simulink model "TP4_control_linealizante_Haldane_params_desconocidos_int"  (R2024b)
settings: Solver=VariableStepAuto  StartTime=0.0  StopTime=10.0  FixedStep=0.  RelTol=1e-3
values from neighbouring files (symbols this model uses):
  e0 = mu_r*1.5    (= 0.12675)    [Main_entregable.m]
  states0 = [x0;s0]*1.5    [DatosModeloTP4.m]    (also in Main_entregable.m = [x0;s0;0;0]*1.5)
  v0 = 1    [DatosModeloTP4.m]
settings Model: Creator=tomii  LastModifiedBy=tomii

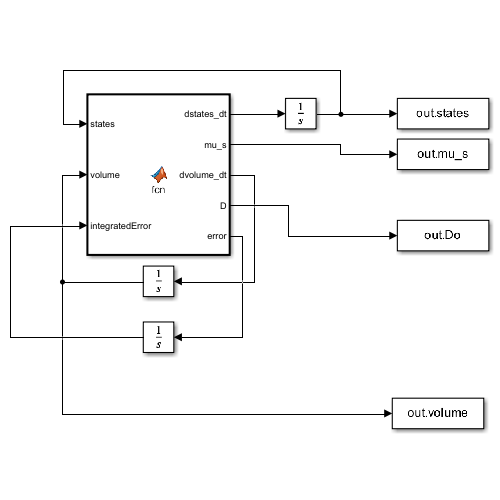
[thumbnail: Simulink's stored preview of the top-level diagram]
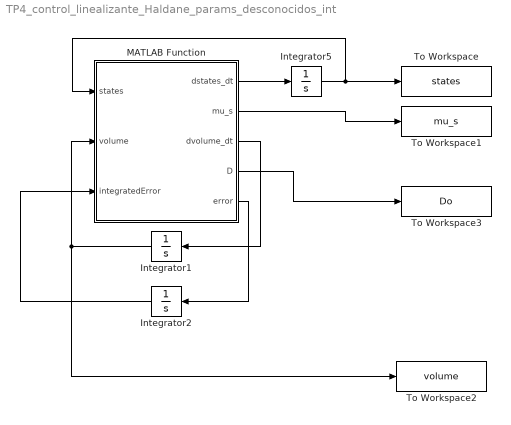
== system TP4_control_linealizante_Haldane_params_desconocidos_int ==
  Integrator1 : Integrator  InitialCondition=v0
  Integrator2 : Integrator  InitialCondition=e0
  Integrator5 : Integrator  InitialCondition=states0
  MATLAB Function : MATLAB Function  TreatAsAtomicUnit=on
  To Workspace : ToWorkspace  VariableName=states  SaveFormat=Timeseries  SampleTime=-1
  To Workspace1 : ToWorkspace  VariableName=mu_s  SaveFormat=Timeseries  SampleTime=-1
  To Workspace2 : ToWorkspace  VariableName=volume  SaveFormat=Timeseries  SampleTime=-1
  To Workspace3 : ToWorkspace  VariableName=Do  SaveFormat=Timeseries  SampleTime=-1
  wires:
  MATLAB Function/1(dstates_dt) -> Integrator5/1
  Integrator5/1 -> MATLAB Function/1(states), To Workspace/1
  MATLAB Function/2(mu_s) -> To Workspace1/1
  MATLAB Function/3(dvolume_dt) -> Integrator1/1
  Integrator1/1 -> MATLAB Function/2(volume), To Workspace2/1
  MATLAB Function/4(D) -> To Workspace3/1
  Integrator2/1 -> MATLAB Function/3(integratedError)
  MATLAB Function/5(error) -> Integrator2/1

== matlab function TP4_control_linealizante_Haldane_params_desconocidos_int/MATLAB Function ==
  data: dstates_dt output; mu_s output; states input; volume input; integratedError input; modelParameters parameter; dvolume_dt output; D output; error output
function [dstates_dt, mu_s, dvolume_dt, D, error] = fcn(states, volume, integratedError, modelParameters)   
    
    K=modelParameters.K;
    xi_in=modelParameters.xi_in;
    mu_r=modelParameters.mu_r;
    s_r=modelParameters.s_r;
    x0=modelParameters.x0;
    s_in=modelParameters.s_in;
    kp=modelParameters.kp;
    ks=modelParameters.ks;
    ki=modelParameters.ki;

    Ks=modelParameters.mu_model.Ks;
    mu_max=modelParameters.mu_model.mu_max;
    Kis=modelParameters.mu_model.Kis;

    x=states(1);
    s=states(2);

    mu_s=mu_max*(s/(s+Ks+s*s/Kis));
    rx=x*mu_s;

    error=s_r-s;
    D=x*(kp*error+ki*integratedError)/(s_in-s);

    dstates_dt = K * rx + D*(xi_in-states);
    dvolume_dt = volume*D;

end
